simulink model "questao01_pat_estimador"  (R2020a)
settings: Solver=VariableStepAuto  StartTime=0.0  StopTime=50  RelTol=1e-3
values from neighbouring files (symbols this model uses):
  A = [1 2 0;-1 -1 -1;0 2 -1]    [lqr_estudos.m]    (also in questao2_pat.m = [1 2 0; -1 -1 -1; 0 2 -1])
  Alc = A - L * C    [questao1_pat.m]    (also in questao2_pat.m)
  B = [0;0;2]    [lqr_estudos.m]    (also in questao2_pat.m)
  C = [0 1 0;0 0 1]    [lqr_estudos.m]    (also in questao2_pat.m = [0 1 0; 0 0 1])
  K = place(A,B,poles)    [estudos_versao_laurinda.m]    (also in lqr_estudos.m = lqr(A,B,Q,R); questao1_pat.m = Ka(1:3); questao1_well.m = Ka(1:3); questao2_pat.m = place(A,B,newpoles))
  Kz = 1    [estudos_versao_laurinda.m]    (also in questao1_pat.m = Ka(4); questao1_well.m = Ka(4))
  L = L'    [questao1_pat.m]    (also in questao2_pat.m)
settings Model: Creator=wwagner  LastModifiedBy=patricia

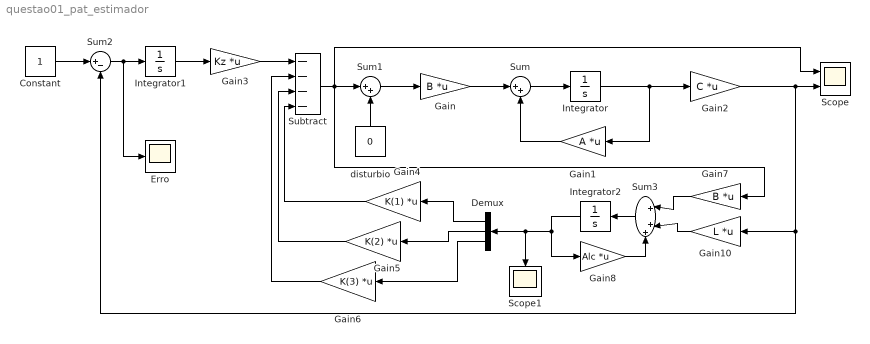
== system questao01_pat_estimador ==
  Constant : Constant
  Demux : Demux  Outputs=3
  Erro : Scope
  Gain : Gain  Gain=B  Multiplication=Matrix(K*u)
  Gain1 : Gain  Gain=A  Multiplication=Matrix(K*u)
  Gain10 : Gain  Gain=L  Multiplication=Matrix(K*u)
  Gain2 : Gain  Gain=C  Multiplication=Matrix(K*u)
  Gain3 : Gain  Gain=Kz  Multiplication=Matrix(K*u)
  Gain4 : Gain  Gain=K(1)  Multiplication=Matrix(K*u)
  Gain5 : Gain  Gain=K(2)  Multiplication=Matrix(K*u)
  Gain6 : Gain  Gain=K(3)  Multiplication=Matrix(K*u)
  Gain7 : Gain  Gain=B  Multiplication=Matrix(K*u)
  Gain8 : Gain  Gain=Alc  Multiplication=Matrix(K*u)
  Integrator : Integrator
  Integrator1 : Integrator
  Integrator2 : Integrator
  Scope : Scope  NumInputPorts=2
  Scope1 : Scope
  Subtract : Sum  Inputs=----
  Sum : Sum  Inputs=|++
  Sum1 : Sum  Inputs=|++
  Sum2 : Sum  Inputs=|+-
  Sum3 : Sum  Inputs=|+++
  disturbio : Constant  Value=0
  wires:
  Integrator/1 -> Gain2/1, Gain1/1
  Gain/1 -> Sum/1
  Gain1/1 -> Sum/2
  Sum/1 -> Integrator/1
  Gain2/1 -> Gain10/1, Sum2/2, Scope/2
  Sum1/1 -> Gain/1
  Sum2/1 -> Erro/1, Integrator1/1
  Constant/1 -> Sum2/1
  Integrator1/1 -> Gain3/1
  Gain3/1 -> Subtract/1
  Subtract/1 -> Gain7/1, Scope/1, Sum1/1
  disturbio/1 -> Sum1/2
  Gain4/1 -> Subtract/4
  Gain5/1 -> Subtract/3
  Gain6/1 -> Subtract/2
  Demux/1 -> Gain4/1
  Demux/2 -> Gain5/1
  Demux/3 -> Gain6/1
  Gain7/1 -> Sum3/1
  Integrator2/1 -> Demux/1, Scope1/1, Gain8/1
  Gain10/1 -> Sum3/2
  Sum3/1 -> Integrator2/1
  Gain8/1 -> Sum3/3
